simulink model "model"  (Simulink 7.7)
settings: Solver=ode45  StartTime=0.0  StopTime=10000  RelTol=1e-3
values from neighbouring files (symbols this model uses):
  fx = exp(1) ^ (-(x ^ 2))    [approximateintegral.m]
settings Model: Creator=ozisoft  LastModifiedBy=ozisoft

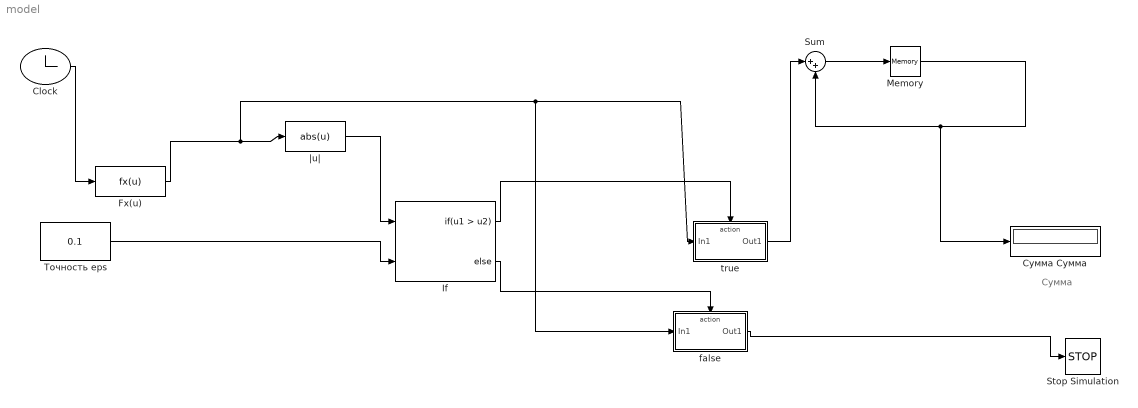
== system model ==
  note: Сумма
  Clock : Clock
  Fx(u) : MATLABFcn  MATLABFcn=fx(u)
  If : If  NumInputs=2  IfExpression=u1 > u2
  Memory : Memory
  Stop Simulation : Stop
  Sum : Sum  Inputs=|++
  false : Subsystem  TreatAsAtomicUnit=on
  true : Subsystem  TreatAsAtomicUnit=on
  |u| : Fcn  Expr=abs(u)
  Сумма Сумма : Display
  Точность eps : Constant  Value=0.1
  wires:
  Clock/1 -> Fx(u)/1
  Fx(u)/1 -> |u|/1, true/1(In1), false/1(In1)
  Точность eps/1 -> If/2
  |u|/1 -> If/1
  If/1 -> true/Action
  true/1(Out1) -> Sum/1
  Sum/1 -> Memory/1
  Memory/1 -> Sum/2, Сумма Сумма/1
  If/2 -> false/Action
  false/1(Out1) -> Stop Simulation/1

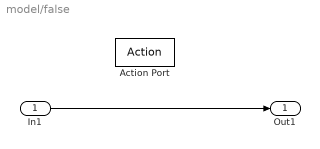
== system model/false ==
  In1 : Inport
  Action Port : ActionPort  ActionType=else
  Out1 : Outport
  wires:
  In1/1 -> Out1/1

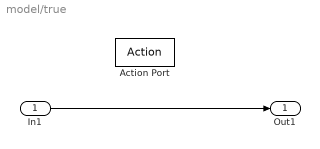
== system model/true ==
  In1 : Inport
  Action Port : ActionPort  ActionType=then
  Out1 : Outport
  wires:
  In1/1 -> Out1/1
